simulink model "CL1CM1"  (R2024a)
settings: Solver=VariableStepAuto  StartTime=0.0  StopTime=10.0  RelTol=1e-3
settings Model: Creator=jeonghyun  LastModifiedBy=gluts

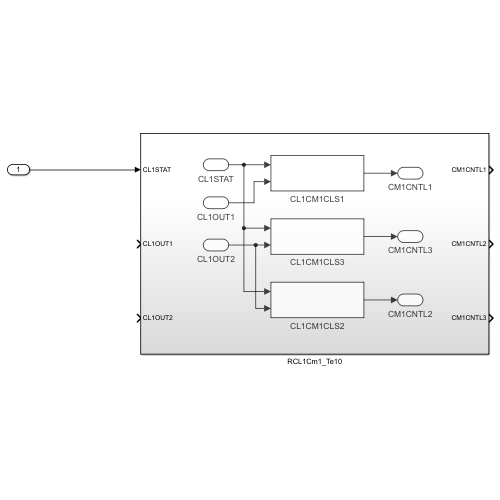
[thumbnail: Simulink's stored preview of the top-level diagram]
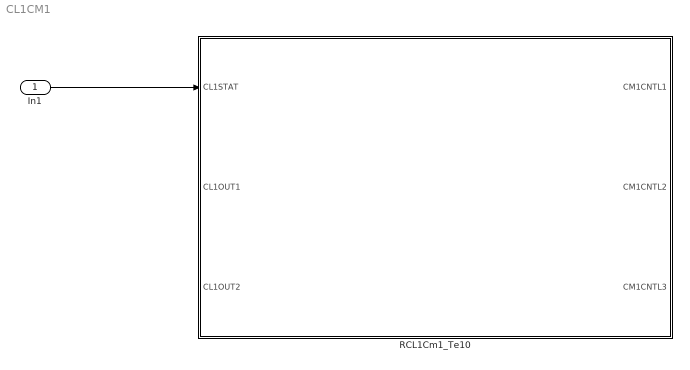
== system CL1CM1 ==
  In1 : Inport
  RCL1Cm1_Te10 : Subsystem
  wires:
  In1/1 -> RCL1Cm1_Te10/1(CL1STAT)

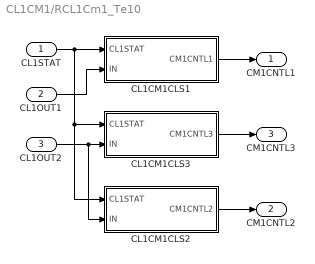
== system CL1CM1/RCL1Cm1_Te10 ==
  CL1STAT : Inport
  CL1OUT1 : Inport  Port=2
  CL1OUT2 : Inport  Port=3
  CL1CM1CLS1 : Subsystem
  CL1CM1CLS2 : Subsystem
  CL1CM1CLS3 : Subsystem
  CM1CNTL1 : Outport
  CM1CNTL2 : Outport  Port=2
  CM1CNTL3 : Outport  Port=3
  wires:
  CL1STAT/1 -> CL1CM1CLS3/1(CL1STAT), CL1CM1CLS2/1(CL1STAT), CL1CM1CLS1/1(CL1STAT)
  CL1CM1CLS2/1(CM1CNTL2) -> CM1CNTL2/1
  CL1CM1CLS3/1(CM1CNTL3) -> CM1CNTL3/1
  CL1OUT1/1 -> CL1CM1CLS1/2(IN)
  CL1CM1CLS1/1(CM1CNTL1) -> CM1CNTL1/1
  CL1OUT2/1 -> CL1CM1CLS2/2(IN), CL1CM1CLS3/2(IN)

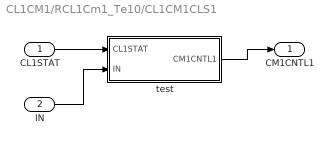
== system CL1CM1/RCL1Cm1_Te10/CL1CM1CLS1 ==
  CL1STAT : Inport
  IN : Inport  Port=2
  test : Subsystem
  CM1CNTL1 : Outport
  wires:
  CL1STAT/1 -> test/1(CL1STAT)
  IN/1 -> test/2(IN)
  test/1(CM1CNTL1) -> CM1CNTL1/1

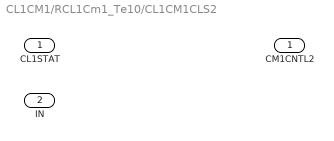
== system CL1CM1/RCL1Cm1_Te10/CL1CM1CLS2 ==
  CL1STAT : Inport
  IN : Inport  Port=2
  CM1CNTL2 : Outport

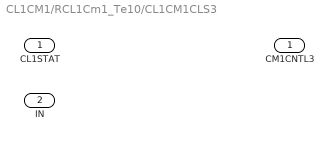
== system CL1CM1/RCL1Cm1_Te10/CL1CM1CLS3 ==
  CL1STAT : Inport
  IN : Inport  Port=2
  CM1CNTL3 : Outport

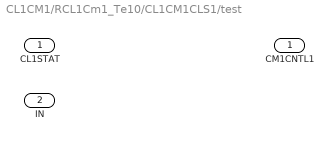
== system CL1CM1/RCL1Cm1_Te10/CL1CM1CLS1/test ==
  CL1STAT : Inport
  IN : Inport  Port=2
  CM1CNTL1 : Outport
